simulink library "commblkintrlv2"  (Simulink 6.0)
settings: Solver=ode45  SolverMode=SingleTasking  StartTime=0.0  StopTime=10.0  RelTol=1e-3
libraries: commblkintrlv2 x8
settings Model: RequirementInfo=9  Creator=mikem  LastModifiedBy=cvora  ExtModeAutoUpdateStatusClock=off
settings DataIOCC: SignalLoggingName=logsOut
settings OptimizationCC: BooleanDataType=off
settings DebuggingCC: CheckExecutionContextPreStartOutputMsg=on  CheckExecutionContextRuntimeOutputMsg=on  SolverPrmCheckMsg=none
settings HardwareCC: TargetUnknown=on
settings SFSimCC: SFSimApplyToAllLibs=on  SFSimBuildMode=Incremental

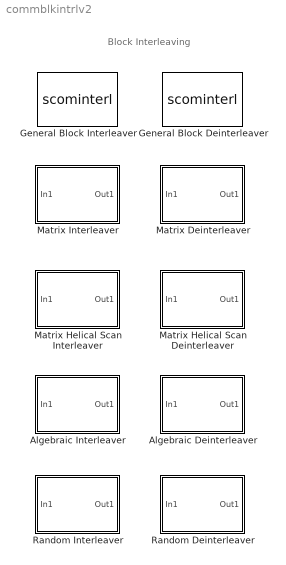
== system commblkintrlv2 ==
  note: Block Interleaving
  Algebraic Deinterleaver : Subsystem  PropExecContextAcrossSSBoundary=on  mask(Algebraic Deinterleaver){intType=Takeshita-Costello, N=256, k=13, h=0, alpha=6}
      mask prompts: intType "Type:"; N "Number of elements:"; k "Multiplicative factor:"; h "Cyclic shift:"; alpha "Primitive element:"
      mask help:
      | Deinterleave the elements of the input vector using an algebraically derived permutation table.
      |
      | For the Takeshita-Costello type interleaver, the Number of elements N must be a power of 2, the Multiplicative factor must be an odd integer less than N, and the Cyclic shift must be a nonnegative integer less than N.
      |
      | For the Welch-Costas type interleaver, the Number of elements N must be specified such that N+1 is prime and the Primitive element must be a primitive element from GF(N+1).
      |
      | In each case, the Number of elements must match the input signal width.
      mask init:
      | int_tb = commblkalgintrlvr(gcb,'init');
      | int_table = int_tb.';
      mask Help: helpview(commbhelp)
      mask StyleString: popup(Takeshita-Costello|Welch-Costas),edit,edit,edit,edit
      mask CallbackString: commblkalgintrlvr(gcb,'Mode');||||
      mask Display: disp('Algebraic\nDeinterleaver')
  Algebraic Interleaver : Subsystem  PropExecContextAcrossSSBoundary=on  mask(Algebraic Interleaver){intType=Takeshita-Costello, N=256, k=13, h=0, alpha=6}
      mask prompts: intType "Type:"; N "Number of elements:"; k "Multiplicative factor:"; h "Cyclic shift:"; alpha "Primitive element:"
      mask help:
      | Interleave the elements of the input vector using an algebraically derived permutation table.
      |
      | For the Takeshita-Costello type interleaver, the Number of elements N must be a power of 2, the Multiplicative factor must be an odd integer less than N, and the Cyclic shift must be a nonnegative integer less than N.
      |
      | For the Welch-Costas type interleaver, the Number of elements N must be specified such that N+1 is prime and the Primitive element must be a primitive element from GF(N+1).
      |
      | In each case, the Number of elements must match the input signal width.
      mask init:
      | int_tb = commblkalgintrlvr(gcb,'init');
      | int_table = int_tb.';
      mask Help: helpview(commbhelp)
      mask StyleString: popup(Takeshita-Costello|Welch-Costas),edit,edit,edit,edit
      mask CallbackString: commblkalgintrlvr(gcb,'Mode');||||
      mask Display: disp('Algebraic\nInterleaver')
  General Block Deinterleaver : S-Function  FunctionName=scominterl  Parameters=elements,method  mask(General Block Deinterleaver){elements=[5:-1:1].'}
      mask help: Reorder the elements of the input vector. y(elements) = u. The length of Elements must match the input signal width.
      mask init:
      | method = 2;
      | commblkinterl(elements);
      mask Help: helpview(commbhelp)
      mask Display: disp('General\nBlock\nDeinterleaver')
  General Block Interleaver : S-Function  FunctionName=scominterl  Parameters=elements,method  mask(General Block Interleaver){elements=[5:-1:1].'}
      mask help: Reorder the elements of the input vector. y = u(Elements). The length of Elements must match the input signal width.
      mask init:
      | method = 1;
      | commblkinterl(elements);
      mask Help: helpview(commbhelp)
      mask Display: disp('General\nBlock\nInterleaver')
  Matrix Deinterleaver : Subsystem  PropExecContextAcrossSSBoundary=on  mask(Matrix Deinterleaver){Nrows=3, Ncols=4}
      mask prompts: Nrows "Number of rows:"; Ncols "Number of columns:"
      mask help: Deinterleave the input vector by writing the elements into a matrix column-by-column and reading them out row-by-row. The product of Number of rows and Number of columns must match the input signal width.
      mask init:
      | int_table = reshape(reshape([1:Nrows*Ncols],Ncols,Nrows)',Nrows*Ncols,1);
      mask Help: helpview(commbhelp)
      mask Display: disp('Matrix\nDeinterleaver')
  Matrix Helical Scan Deinterleaver : Subsystem  PropExecContextAcrossSSBoundary=on  mask(Matrix helical scan deinterleaver){Nrows=64, Ncols=64, Hstep=1}
      mask prompts: Nrows "Number of rows:"; Ncols "Number of columns:"; Hstep "Array step size:"
      mask help:
      | Restore the ordering of symbols permuted by a matching helical scan interleaver.  The helical scan interleaver writes input elements row-by-row into an array with a specified number of rows and columns.  The interleaver output is then read by scanning along diagonals of this array.  The pitch of the diagonal scans is determined by the array step size.
      |
      | The array step size must be a nonnegative integer less than the specified number of rows.  An array step size of zero indicates no interleaving.
      |
      | The product of Number of rows and Number of columns must match the input signal width.
      mask init:
      | if(Nrows<=0)
      |    error('The number of rows must be a nonnegative integer.');
      | end
      | 
      | if(Ncols<=0)
      |    error('The number of columns must be a nonnegative integer.');
      | end
      | 
      | if Hstep>=Nrows | Hstep<0
      |     error('The array step size must be a nonnegative integer less than the specified number of rows.');
      | end
      | 
      | int_table = zeros(Nrows*Ncols,1);
      | for i=1:Nrows
      |  j=1:Ncols;
      |  int_table((i-1)*Ncols+j)=mod(i-1+Hstep*(j-1),Nrows)*Ncols+j;
      | end
      mask Help: helpview(commbhelp)
      mask Display: disp('Matrix\nHelical Scan\nDeinterleaver')
  Matrix Helical Scan Interleaver : Subsystem  PropExecContextAcrossSSBoundary=on  mask(Matrix helical scan interleaver){Nrows=64, Ncols=64, Hstep=1}
      mask prompts: Nrows "Number of rows:"; Ncols "Number of columns:"; Hstep "Array step size:"
      mask help:
      | Interleave input vector by writing elements row-by-row into an array with a specified number of rows and columns and then reading them out by scanning along diagonals of this array.  The pitch of the diagonal scans is determined by the array step size.
      |
      | The array step size must be a nonnegative integer less than the specified number of rows.  An array step size of zero indicates no interleaving.
      |
      | The product of Number of rows and Number of columns must match the input signal width.
      mask init:
      | if(Nrows<=0)
      |    error('The number of rows must be a nonnegative integer.');
      | end
      | 
      | if(Ncols<=0)
      |    error('The number of columns must be a nonnegative integer.');
      | end
      | 
      | if Hstep>=Nrows | Hstep<0
      |     error('The array step size must be a nonnegative integer less than the specified number of rows.');
      | end
      | 
      | int_table = zeros(Nrows*Ncols,1);
      | for i=1:Nrows
      |  j=1:Ncols;
      |  int_table((i-1)*Ncols+j)=mod(i-1+Hstep*(j-1),Nrows)*Ncols+j;
      | end
      mask Help: helpview(commbhelp)
      mask Display: disp('Matrix\nHelical Scan\nInterleaver')
  Matrix Interleaver : Subsystem  PropExecContextAcrossSSBoundary=on  mask(Matrix Interleaver){Nrows=3, Ncols=4}
      mask prompts: Nrows "Number of rows:"; Ncols "Number of columns:"
      mask help: Interleave the input vector by writing the elements into a matrix row-by-row and reading them out column-by-column. The product of Number of rows and Number of columns must match the input signal width.
      mask init:
      | int_table = reshape(reshape([1:Nrows*Ncols],Ncols,Nrows)',Nrows*Ncols,1);
      mask Help: helpview(commbhelp)
      mask Display: disp('Matrix\nInterleaver')
  Random Deinterleaver : Subsystem  PropExecContextAcrossSSBoundary=on  mask(Random Deinterleaver){N=100, seed=12345}
      mask prompts: N "Number of elements:"; seed "Initial seed:"
      mask help: Deinterleave the elements of the input vector using a random permutation. The Number of elements must match the input signal width.
      mask init:
      | rand('state',seed);
      | int_table = (randperm(N)).';
      mask Help: helpview(commbhelp)
      mask Display: disp('Random\nDeinterleaver')
  Random Interleaver : Subsystem  PropExecContextAcrossSSBoundary=on  mask(Random Interleaver){N=100, seed=12345}
      mask prompts: N "Number of elements:"; seed "Initial seed:"
      mask help: Interleave the elements of the input vector using a random permutation. The Number of elements must match the input signal width.
      mask init:
      | rand('state',seed);
      | int_table = (randperm(N)).';
      mask Help: helpview(commbhelp)
      mask Display: disp('Random\nInterleaver')

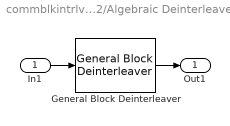
== system commblkintrlv2/Algebraic Deinterleaver ==
  In1 : Inport  LatchInput=off
  General Block Deinterleaver : commblkintrlv2/General Block Deinterleaver  elements=int_table
  Out1 : Outport
  wires:
  In1/1 -> General Block Deinterleaver/1
  General Block Deinterleaver/1 -> Out1/1

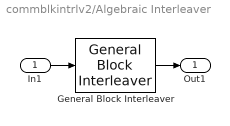
== system commblkintrlv2/Algebraic Interleaver ==
  In1 : Inport  LatchInput=off
  General Block Interleaver : commblkintrlv2/General Block Interleaver  elements=int_table
  Out1 : Outport
  wires:
  General Block Interleaver/1 -> Out1/1
  In1/1 -> General Block Interleaver/1

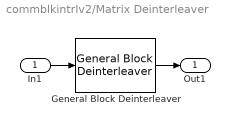
== system commblkintrlv2/Matrix Deinterleaver ==
  In1 : Inport  LatchInput=off
  General Block Deinterleaver : commblkintrlv2/General Block Deinterleaver  elements=int_table
  Out1 : Outport
  wires:
  General Block Deinterleaver/1 -> Out1/1
  In1/1 -> General Block Deinterleaver/1

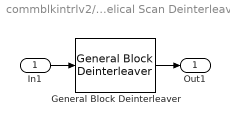
== system commblkintrlv2/Matrix Helical Scan Deinterleaver ==
  In1 : Inport  LatchInput=off
  General Block Deinterleaver : commblkintrlv2/General Block Deinterleaver  elements=int_table
  Out1 : Outport
  wires:
  General Block Deinterleaver/1 -> Out1/1
  In1/1 -> General Block Deinterleaver/1

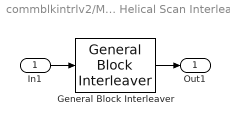
== system commblkintrlv2/Matrix Helical Scan Interleaver ==
  In1 : Inport  LatchInput=off
  General Block Interleaver : commblkintrlv2/General Block Interleaver  elements=int_table
  Out1 : Outport
  wires:
  In1/1 -> General Block Interleaver/1
  General Block Interleaver/1 -> Out1/1

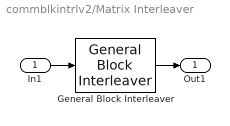
== system commblkintrlv2/Matrix Interleaver ==
  In1 : Inport  LatchInput=off
  General Block Interleaver : commblkintrlv2/General Block Interleaver  elements=int_table
  Out1 : Outport
  wires:
  In1/1 -> General Block Interleaver/1
  General Block Interleaver/1 -> Out1/1

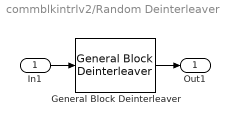
== system commblkintrlv2/Random Deinterleaver ==
  In1 : Inport  LatchInput=off
  General Block Deinterleaver : commblkintrlv2/General Block Deinterleaver  elements=int_table
  Out1 : Outport
  wires:
  In1/1 -> General Block Deinterleaver/1
  General Block Deinterleaver/1 -> Out1/1

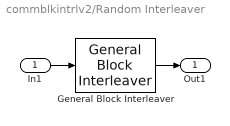
== system commblkintrlv2/Random Interleaver ==
  In1 : Inport  LatchInput=off
  General Block Interleaver : commblkintrlv2/General Block Interleaver  elements=int_table
  Out1 : Outport
  wires:
  General Block Interleaver/1 -> Out1/1
  In1/1 -> General Block Interleaver/1
